simulink model "derivace_RL"  (R2021a)
settings: Solver=VariableStepAuto  StartTime=0.0  StopTime=0.2e-3  RelTol=1e-3
undefined symbols (not defined in the file): L, R, U_0
settings Model: Creator=vojte  LastModifiedBy=vojte

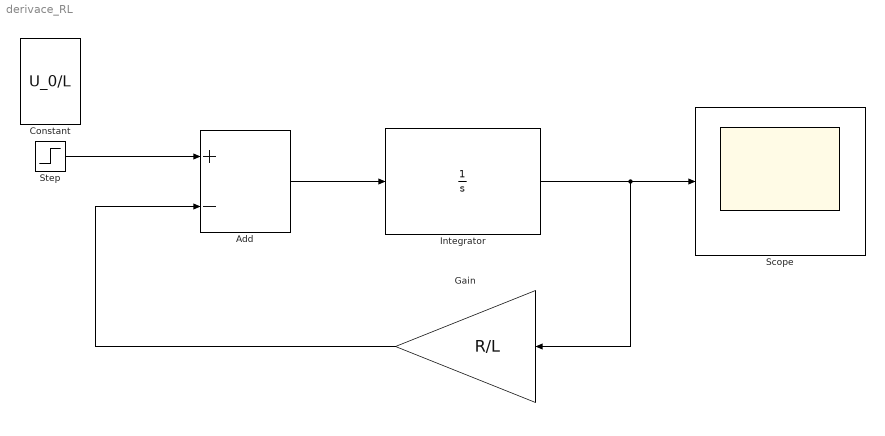
== system derivace_RL ==
  Add : Sum  Inputs=+-
  Constant : Constant  Value=U_0/L
  Gain : Gain  Gain=R/L
  Integrator : Integrator
  Scope : Scope
  Step : Step  Time=0.1e-3  Before=U_0/L  After=0  SampleTime=0
  wires:
  Add/1 -> Integrator/1
  Integrator/1 -> Scope/1, Gain/1
  Gain/1 -> Add/2
  Step/1 -> Add/1
